simulink subsystem "block_admittance_controller_euler"  (R2021b)
settings: Solver=VariableStepAuto  StartTime=0.0  StopTime=10.0  RelTol=1e-3
undefined symbols (not defined in the file): dphi_cd0, Kd, Kp, Md, phi_cd0
settings Model: Creator=Martin  LastModifiedBy=Martin

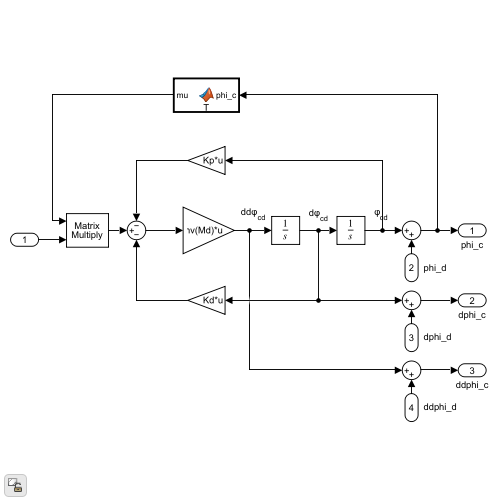
[thumbnail: Simulink's stored preview of the top-level diagram]
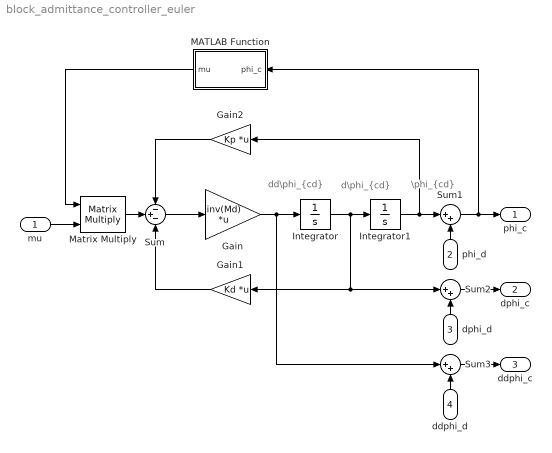
== system block_admittance_controller_euler ==
  note: \phi_{cd}
  note: d\phi_{cd}
  note: dd\phi_{cd}
  mu : Inport  PortDimensions=[3 1]
  phi_d : Inport  Port=2  PortDimensions=[3 1]
  dphi_d : Inport  Port=3  PortDimensions=[3 1]
  ddphi_d : Inport  Port=4  PortDimensions=[3 1]
  Gain : Gain  Gain=inv(Md)  Multiplication=Matrix(K*u)
  Gain1 : Gain  Gain=Kd  Multiplication=Matrix(K*u)
  Gain2 : Gain  Gain=Kp  Multiplication=Matrix(K*u)
  Integrator : Integrator  InitialCondition=dphi_cd0
  Integrator1 : Integrator  InitialCondition=phi_cd0
  MATLAB Function : MATLAB Function  TreatAsAtomicUnit=on
  Matrix Multiply : Product  Multiplication=Matrix(*)
  Sum : Sum  Inputs=-+-
  Sum1 : Sum  Inputs=|++
  Sum2 : Sum  Inputs=|++
  Sum3 : Sum  Inputs=|++
  phi_c : Outport
  dphi_c : Outport  Port=2
  ddphi_c : Outport  Port=3
  wires:
  Sum2/1 -> dphi_c/1
  Sum3/1 -> ddphi_c/1
  Integrator/1 -> Integrator1/1, Sum2/1, Gain1/1
  Integrator1/1 -> Gain2/1, Sum1/1
  dphi_d/1 -> Sum2/2
  Gain/1 -> Integrator/1, Sum3/1
  ddphi_d/1 -> Sum3/2
  Sum1/1 -> phi_c/1, MATLAB Function/1(phi_c)
  phi_d/1 -> Sum1/2
  Sum/1 -> Gain/1
  Gain2/1 -> Sum/1
  Gain1/1 -> Sum/3
  MATLAB Function/1(mu) -> Matrix Multiply/1
  mu/1 -> Matrix Multiply/2
  Matrix Multiply/1 -> Sum/2

== matlab function block_admittance_controller_euler/MATLAB Function ==
  data: phi_c input; mu output
function mu = T(phi_c)

    phi = phi_c(1); th = phi_c(2); psi = phi_c(3);

    dphi_ = eye(3); dphi_ = dphi_(:, 1);
    dth_  = eye(3) * rotx(phi); dth_ = dth_(:, 2);
    dpsi_ = eye(3) * rotx(phi) * roty(th); dpsi_ = dpsi_(:, 3);
    
    mu = [dphi_ dth_ dpsi_];
    
end
